simulink model "Vehicle_Model_999_Modular_roll_gradient"  (R2025b)
settings: Solver=ode23tb  StartTime=0.0  StopTime=30  MaxStep=0.001  RelTol=1e-3
values from neighbouring files (symbols this model uses):
  init_r = 0    [Run_this_first.m]
  init_vx = 0    [Run_this_first.m]
  init_vy = 0    [Run_this_first.m]
  Ki_array = zeros(size(Vx_array))    [Torque_vectoring_lookup_table_v3.m]    (also in Torque_vectoring_workspace_lookuptable_v2.m)
  Kp_array = zeros(size(Vx_array))    [Torque_vectoring_workspace_lookuptable_v2.m]
  ku = (lr*m/(cf*(lf+lr))) - (lf*m/(cr*(lf+lr)))    (= -0.000176093739153)    [Torque_vectoring_lookup_table_v3.m]    (also in Torque_vectoring_workspace_lookuptable_v2.m)
  m = Par.m    [LapSim_Endurance_final_ts_v2.m]    (also in Lap_Sim_Final_inverse.m = Par.Mass; Lapsim_Endurance_final_ts.m; New_LapSim_final_ts_v1.m = Par.Mass; Torque_vectoring_lookup_table_v3.m = 270)
  Par = struct()    [Load_vehicle_parameters.m]
  path_Theta = unwrap(atan2(dY, dX))    [New_LapSim_final_ts_v1.m]
  sus_par = struct()    [Load_sus_parameters.m]
  TireData = []    [Lapsim_final_for_app.m]
  V_ref = 45    [Run_this_first.m]
  Vx_array = 1:2:21    [Torque_vectoring_lookup_table_v3.m]    (also in Torque_vectoring_workspace_lookuptable_v2.m = 1:1:21)
undefined symbols (not defined in the file or in its folder): Battery, Brake_Val, ctrl_Brake, ctrl_s, ctrl_Steer, ctrl_Throttle, ctrl_Velocity, HP, Motor, path_X, path_Y, steer_input, Steer_Val, TC_target_slip, Throttle_Val
libraries: simulink x9, autolibshared x3, simulink_extras x2, BatteryEstimators x1
(part 1 of 4)
settings Model: PauseTimes=2  PacingRate=0.001000  Creator=vishal bhujbal  LastModifiedBy=vishal bhujbal
settings SolverCC: ZeroCrossAlgorithm=Adaptive
settings DebuggingCC: AlgebraicLoopMsg=none  IgnoredZcDiagnostic=none

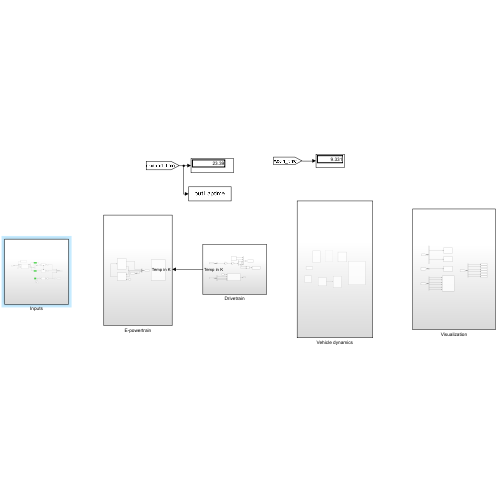
[thumbnail: Simulink's stored preview of the top-level diagram]
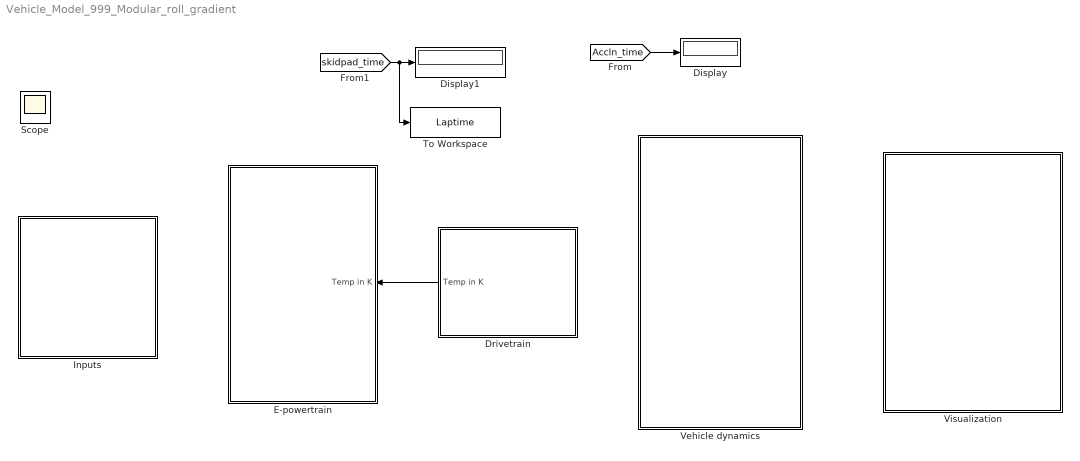
== system Vehicle_Model_999_Modular_roll_gradient ==
  Display : Display
  Display1 : Display
  Drivetrain : Subsystem
      settings: PortSchema="{\"entries\":[{\"content\":{\"sides\":[{\"content\":{\"connectorIds\":[\"Out1\"]},\"type\":\"ConnectorPlacement.EquallySpacedRectSide\",\"uuid\":\"f91cf200-6219-4a1f-80fc-b884c938b97c\"},{\"content\":{\"side\":\"RIGHT\"},\"type\":\"ConnectorPlacement.EquallySpacedRectSide\",\"uuid\":\"1ef2f2a3-0f7e-4e07-a3c9-4fbc06387d99\"},{\"content\":{\"side\":\"TOP\"},\"type\":\"ConnectorPlacement.EquallySpacedRectSide\",\"uuid\":\"4c772986-3ff5-4393-833e-99a2f9c9a16c\"}]},\"type\":\"ConnectorPlacement.EquallySpacedConnector\",\"uuid\":\"ee383106-a54d-4e3a-9b59-9d3772818309\"}],\"packageUris\":[\"http://schema.mathworks.com/mf0/Connector/R2020b\"],\"version\":\"1.0\"}"
  E-powertrain : Subsystem
      settings: PortSchema="{\"entries\":[{\"content\":{\"sides\":[{\"content\":{},\"type\":\"ConnectorPlacement.EquallySpacedRectSide\",\"uuid\":\"2fbe1a29-d7e0-46b2-8acf-c3c60596dfc1\"},{\"content\":{\"connectorIds\":[\"In1\"],\"side\":\"RIGHT\"},\"type\":\"ConnectorPlacement.EquallySpacedRectSide\",\"uuid\":\"5e79f07f-e655-4956-8ef7-fa1f6819f89c\"},{\"content\":{\"side\":\"TOP\"},\"type\":\"ConnectorPlacement.EquallySpacedRectSide\",\"uuid\":\"1ad69596-8b46-43d7-b59f-7fdc3ee385c3\"}]},\"type\":\"ConnectorPlacement.EquallySpacedConnector\",\"uuid\":\"13a1ddb3-f917-41b3-84b0-bd7fb91c78c5\"}],\"packageUris\":[\"http://schema.mathworks.com/mf0/Connector/R2020b\"],\"version\":\"1.0\"}"
  Inputs : Subsystem
  To Workspace : ToWorkspace  VariableName=Laptime  SaveFormat=Timeseries  SampleTime=-1
  Vehicle dynamics : Subsystem
  Visualization : Subsystem
  Scope : Scope
      settings: ActiveDisplayYMinimum=-5.6819269348628578E-5  ActiveDisplayYMaximum=6.3132521498476184E-6  DataLoggingVariableName=ScopeData7
  wires:
  Drivetrain/1(Temp in K) -> E-powertrain/1(Temp in K)
  [Accln_time] -> Display/1
  [skidpad_time] -> To Workspace/1, Display1/1

== system Vehicle_Model_999_Modular_roll_gradient/Drivetrain ==
  Add : Sum
  Bus Selector : BusSelector  OutputSignals=SoC,Omega,I_dc
  Bus Selector1 : BusSelector  OutputSignals=Motor_torque
  Constant : Constant  Value=298
  Demux : Demux  Outputs=2
  Gear Ratio : Gain  Gain=Motor.gear_ratio
  MATLAB Function : MATLAB Function  TreatAsAtomicUnit=on
  Mux : Mux
  Overall Powertrain Efficiency : Gain  Gain=Motor.overall_efficiency
  Thermal : Subsystem
  To Workspace : ToWorkspace  VariableName=Total_wheel_torque  SaveFormat=Timeseries  SampleTime=-1
  Temp in K : Outport
  tag scope: Wheel_torques=global
  wires:
  Bus Selector1/1 -> Gear Ratio/1  "<Motor_torque>"
  Gear Ratio/1 -> Overall Powertrain Efficiency/1
  MATLAB Function/1(T_fl) -> Mux/1
  MATLAB Function/2(T_fr) -> Mux/2
  Demux/1 -> Add/1, Mux/3
  Demux/2 -> Add/2, Mux/4
  Mux/1 -> [Wheel_torques]
  Overall Powertrain Efficiency/1 -> Demux/1
  Thermal/1(Temp in K) -> Temp in K/1
  [Motor_bus] -> Bus Selector/1
  Bus Selector/1 -> Thermal/2(SoC)  "<SoC>"
  Bus Selector/2 -> Thermal/3(Motor speed)  "<Omega>"
  Bus Selector/3 -> Thermal/4(I_dc)  "<I_dc>"
  Constant/1 -> Thermal/1(Ambient Temp)
  [Motor_bus] -> Bus Selector1/1
  Add/1 -> To Workspace/1

== system Vehicle_Model_999_Modular_roll_gradient/E-powertrain ==
  Temp in K : Inport
  Battery Pack : Subsystem
      settings: PortSchema="{\"entries\":[{\"content\":{\"sides\":[{\"content\":{\"connectorIds\":[\"In1\",\"Out2\",\"In2\"]},\"type\":\"ConnectorPlacement.EquallySpacedRectSide\",\"uuid\":\"a12b09be-87e3-41a8-9cce-cb6644b5ba86\"},{\"content\":{\"connectorIds\":[\"Out1\"],\"side\":\"RIGHT\"},\"type\":\"ConnectorPlacement.EquallySpacedRectSide\",\"uuid\":\"19bc61ba-c6fa-40ce-bed9-9c9078ba9fa2\"},{\"content\":{\"side\":\"TOP\"},\"type\":\"ConnectorPlacement.EquallySpacedRectSide\",\"uuid\":\"764d1c28-9cba-450b-a0fd-2f7d4cb2b59a\"}]},\"type\":\"ConnectorPlacement.EquallySpacedConnector\",\"uuid\":\"5b2b37a7-d27f-4738-b8eb-71ceac25d5fc\"}],\"packageUris\":[\"http://schema.mathworks.com/mf0/Connector/R2020b\"],\"version\":\"1.0\"}"
  Bus Creator : BusCreator  Inputs=4
  Bus Selector4 : BusSelector  OutputSignals=Omega
  Motor : Subsystem
  Torque Distribution : Subsystem
  tag scope: Motor_bus=global
  wires:
  Battery Pack/1(V_dc) -> Motor/1(v_dc)
  Motor/1(Motor Torque) -> Bus Creator/1  "Motor_torque"
  Motor/2(I_dc) -> Bus Creator/2, Battery Pack/1(I_dc)  "I_dc"
  Temp in K/1 -> Battery Pack/2(Temp in K)
  Battery Pack/2(SoC) -> Bus Creator/3  "SoC"
  Bus Creator/1 -> [Motor_bus]
  [Wheel_bus] -> Bus Selector4/1
  Bus Selector4/1 -> Bus Creator/4  "<Omega>"

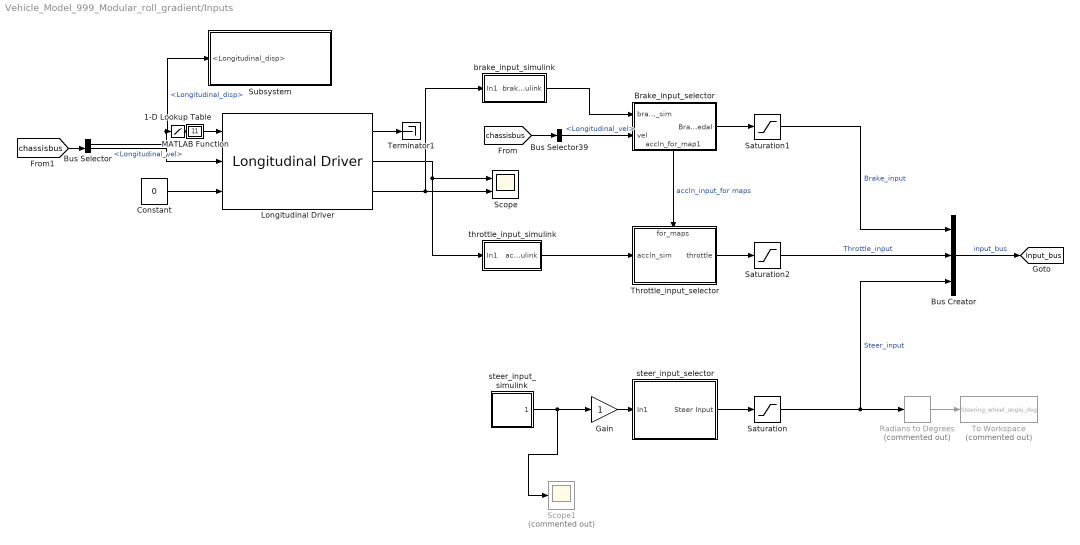
== system Vehicle_Model_999_Modular_roll_gradient/Inputs ==
  1-D Lookup Table : Lookup_n-D  NumberOfTableDimensions=1  BreakpointsForDimension1=ctrl_s  Table=ctrl_Velocity  InternalRulePriority=Speed  RndMeth=Simplest
  Brake_input_selector : Subsystem
      settings: PortSchema="{\"entries\":[{\"content\":{\"sides\":[{\"content\":{\"connectorIds\":[\"In1\",\"In2\"]},\"type\":\"ConnectorPlacement.EquallySpacedRectSide\",\"uuid\":\"eae5282b-8d4e-4a76-acd5-b309529286e8\"},{\"content\":{\"connectorIds\":[\"Out1\"],\"side\":\"RIGHT\"},\"type\":\"ConnectorPlacement.EquallySpacedRectSide\",\"uuid\":\"e88b1ae5-ebac-4dec-84e3-4990dfef2a20\"},{\"content\":{\"side\":\"TOP\"},\"type\":\"ConnectorPlacement.EquallySpacedRectSide\",\"uuid\":\"953e68b4-cb24-4ebf-9e87-e8908532a5e9\"},{\"content\":{\"connectorIds\":[\"Out2\"],\"side\":\"BOTTOM\"},\"type\":\"ConnectorPlacement.EquallySpacedRectSide\",\"uuid\":\"cb4e4aaa-ddd9-4948-8132-cd5bc6a16c6f\"}]},\"type\":\"ConnectorPlacement.EquallySpacedConnector\",\"uuid\":\"c57fd576-21a2-411a-8f11-bf01f4b27bc3\"}],\"packageUris\":[\"http://schema.mathworks.com/mf0/Connector/R2020b\"],\"version\":\"1.0\"}"
  Bus Creator : BusCreator  Inputs=3
  Bus Selector : BusSelector  OutputSignals=Longitudinal_disp,Longitudinal_vel
  Bus Selector39 : BusSelector  OutputSignals=Longitudinal_vel
  Constant : Constant  Value=0
  Gain : Gain
  Longitudinal Driver : autolibshared/Longitudinal Driver  extAccelOvr=off  extDecelOvr=off  extAccelHld=off  extDecelHld=off  extAccelZero=off  extDecelZero=off  cntrlType=PI  shftType=None  velUnits=m/s  gearOut=off  Kp=13.2353  Ki=5.00045  Kff=0.15  Kg=0  VehVelVec=[0 100]  KffVec=[.1 .1]  KpVec=[10 10]  KiVec=[5 5]  KgVec=[0 0]  m=1500  Kpt=3000  tau=.1  L=2  aR=200  bR=2.5  cR=.5  g=9.81  vnom=5  Kaw=1  tauerr=.01  tauPt=2  GearInit=0  tShift=.1  pdlVec=[0.1 0.4 0.5 0.9]  upShftTbl=[-1 12.9375 26.4375 39.9375 51.18749999999999 62.4375 72.84375 83.25;-1 16.3125 29.8125 43.3125 54.5624 65.8125 76.78125 87.75;-1 19.6875 33.1875 46.68749999999999 57.9375 69.1875 80.71875 92.25;-1 33 52.5 77.25 100.5 138.75 161.875 185]  dwnShftTbl=[1 9.5625 23.0625 36.5625 47.8125 59.0625 68.90625 78.75;1 12.9375 26.4375 39.9375 51.18749999999999 62.4375 72.84375 83.25;1 16.3125 29.8125 43.3125 54.562499 65.8125 76.78125 87.75;1 19.6875 33.1875 46.68749999999999 57.9375 69.1875 80.71875 92.25]  tClutch=.5  tRev=.5  tPark=120  aMode=2  UpGearVec="[0  1  2  3  4  5  6  7]"  DownGearVec="[1  2  3  4  5  6  7  8]"
      settings: LibrarySourceBlock=vehdynlibdriver/Longitudinal Driver
  MATLAB Function : MATLAB Function  TreatAsAtomicUnit=on
  Radians to Degrees : simulink_extras/Transformations/Radians to Degrees  Commented=on
  Saturation : Saturate  UpperLimit=pi/6  LowerLimit=-pi/6
  Saturation1 : Saturate  UpperLimit=1  LowerLimit=0
  Saturation2 : Saturate  UpperLimit=1  LowerLimit=0
  Scope : Scope  NumInputPorts=2
      settings: ActiveDisplayYMinimum=-0.12499999999999997  ActiveDisplayYMaximum=1.125  DataLoggingVariableName=ScopeData9
  Scope1 : Scope  Commented=on
      settings: ActiveDisplayYMinimum=-0.21672639126737681  ActiveDisplayYMaximum=0.21672588045733382  DataLoggingVariableName=ScopeData14
  Subsystem : Subsystem
  Terminator1 : Terminator
  Throttle_input_selector : Subsystem
      settings: PortSchema="{\"entries\":[{\"content\":{\"sides\":[{\"content\":{\"connectorIds\":[\"In1\"]},\"type\":\"ConnectorPlacement.EquallySpacedRectSide\",\"uuid\":\"91e59d49-26fd-4266-b297-7cd1b1ce02c9\"},{\"content\":{\"connectorIds\":[\"Out1\"],\"side\":\"RIGHT\"},\"type\":\"ConnectorPlacement.EquallySpacedRectSide\",\"uuid\":\"6279f554-8ceb-423b-aff4-2d71feb4a43a\"},{\"content\":{\"connectorIds\":[\"In2\"],\"side\":\"TOP\"},\"type\":\"ConnectorPlacement.EquallySpacedRectSide\",\"uuid\":\"41f52c32-a07b-4398-ae75-202afa1bbaca\"}]},\"type\":\"ConnectorPlacement.EquallySpacedConnector\",\"uuid\":\"9d03091e-cc24-4a85-a828-51493ad70cf1\"}],\"packageUris\":[\"http://schema.mathworks.com/mf0/Connector/R2020b\"],\"version\":\"1.0\"}"
  To Workspace : ToWorkspace  Commented=on  VariableName=Steering_wheel_angle_deg  SaveFormat=Timeseries  SampleTime=-1
  brake_input_simulink : Subsystem
  steer_input_selector : Subsystem
  steer_input_simulink : Subsystem
  throttle_input_simulink : Subsystem
  tag scope: Input_bus=global
  wires:
  Throttle_input_selector/1(throttle) -> Saturation2/1
  throttle_input_simulink/1(accln_simulink) -> Throttle_input_selector/1(accln_sim)
  Brake_input_selector/2(accln_for_map1) -> Throttle_input_selector/2(for_maps)  "accln_input_for maps"
  Bus Selector39/1 -> Brake_input_selector/2(vel)  "<Longitudinal_vel>"
  Brake_input_selector/1(Brake pedal) -> Saturation1/1
  brake_input_simulink/1(brake_simulink) -> Brake_input_selector/1(brake_sim)
  steer_input_simulink/1(cmd_str) -> Scope1/1, Gain/1
  steer_input_selector/1(Steer Input) -> Saturation/1
  Bus Creator/1 -> [Input_bus]  "input_bus"
  Saturation/1 -> Radians to Degrees/1, Bus Creator/3  "Steer_input"
  Saturation1/1 -> Bus Creator/1  "Brake_input"
  Saturation2/1 -> Bus Creator/2  "Throttle_input"
  [chassisbus] -> Bus Selector39/1
  Radians to Degrees/1 -> To Workspace/1
  [chassisbus] -> Bus Selector/1
  Bus Selector/2 -> Longitudinal Driver/2  "<Longitudinal_vel>"
  Constant/1 -> Longitudinal Driver/3
  Bus Selector/1 -> Subsystem/1(<Longitudinal_disp>), 1-D Lookup Table/1  "<Longitudinal_disp>"
  Longitudinal Driver/2 -> throttle_input_simulink/1(In1), Scope/1
  Longitudinal Driver/1 -> Terminator1/1
  MATLAB Function/1(y) -> Longitudinal Driver/1
  Longitudinal Driver/3 -> brake_input_simulink/1(In1), Scope/2
  Gain/1 -> steer_input_selector/1(In1)
  1-D Lookup Table/1 -> MATLAB Function/1(ideal_ref_vel)

== system Vehicle_Model_999_Modular_roll_gradient/Vehicle dynamics ==
  Brakes : Subsystem
  Force and Torque Equilibrium : Subsystem
  "Fx, Fy calculations" : Subsystem  Commented=on
  "Fx, Fy calculations with grip limit" : Subsystem
  Rolling and Drag forces : Subsystem
  Steering : Subsystem
  Suspension : Subsystem
  Wheel_dynamics : Subsystem
  wires:
  Wheel_dynamics/1(Omega1) -> Suspension/1(Omega)

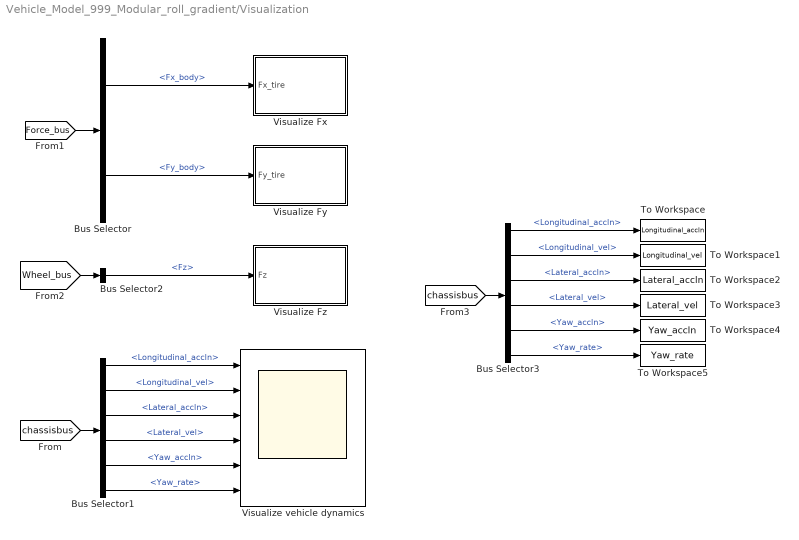
== system Vehicle_Model_999_Modular_roll_gradient/Visualization ==
  Bus Selector : BusSelector  OutputSignals=Fx_body,Fy_body
  Bus Selector1 : BusSelector  OutputSignals=Longitudinal_accln,Longitudinal_vel,Lateral_accln,Lateral_vel,Yaw_accln,Yaw_rate
  Bus Selector2 : BusSelector  OutputSignals=Fz
  Bus Selector3 : BusSelector  OutputSignals=Longitudinal_accln,Longitudinal_vel,Lateral_accln,Lateral_vel,Yaw_accln,Yaw_rate
  To Workspace : ToWorkspace  VariableName=Longitudinal_accln  SaveFormat=Timeseries  SampleTime=-1
  To Workspace1 : ToWorkspace  VariableName=Longitudinal_vel  SaveFormat=Timeseries  SampleTime=-1
  To Workspace2 : ToWorkspace  VariableName=Lateral_accln  SaveFormat=Timeseries  SampleTime=-1
  To Workspace3 : ToWorkspace  VariableName=Lateral_vel  SaveFormat=Timeseries  SampleTime=-1
  To Workspace4 : ToWorkspace  VariableName=Yaw_accln  SaveFormat=Timeseries  SampleTime=-1
  To Workspace5 : ToWorkspace  VariableName=Yaw_rate  SaveFormat=Timeseries  SampleTime=-1
  Visualize Fx : Subsystem
  Visualize Fy : Subsystem
  Visualize Fz : Subsystem
  Visualize vehicle dynamics : Scope  NumInputPorts=6
      settings: ActiveDisplayYMinimum=-11.262828862578662  ActiveDisplayYMaximum=8.2206676714982336
  wires:
  [Force_bus] -> Bus Selector/1
  [chassisbus] -> Bus Selector1/1
  Bus Selector1/1 -> Visualize vehicle dynamics/1  "<Longitudinal_accln>"
  Bus Selector1/2 -> Visualize vehicle dynamics/2  "<Longitudinal_vel>"
  Bus Selector1/3 -> Visualize vehicle dynamics/3  "<Lateral_accln>"
  Bus Selector1/4 -> Visualize vehicle dynamics/4  "<Lateral_vel>"
  Bus Selector1/5 -> Visualize vehicle dynamics/5  "<Yaw_accln>"
  Bus Selector/1 -> Visualize Fx/1(Fx_tire)  "<Fx_body>"
  [Wheel_bus] -> Bus Selector2/1
  Bus Selector2/1 -> Visualize Fz/1(Fz)  "<Fz>"
  Bus Selector3/5 -> To Workspace4/1  "<Yaw_accln>"
  Bus Selector3/4 -> To Workspace3/1  "<Lateral_vel>"
  Bus Selector3/3 -> To Workspace2/1  "<Lateral_accln>"
  Bus Selector3/2 -> To Workspace1/1  "<Longitudinal_vel>"
  Bus Selector3/1 -> To Workspace/1  "<Longitudinal_accln>"
  [chassisbus] -> Bus Selector3/1
  Bus Selector/2 -> Visualize Fy/1(Fy_tire)  "<Fy_body>"
  Bus Selector3/6 -> To Workspace5/1  "<Yaw_rate>"
  Bus Selector1/6 -> Visualize vehicle dynamics/6  "<Yaw_rate>"

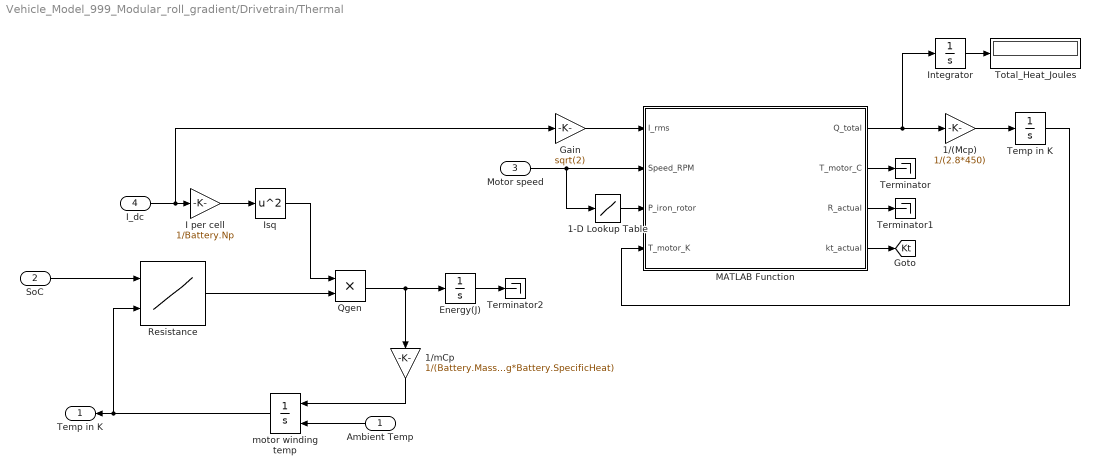
== system Vehicle_Model_999_Modular_roll_gradient/Drivetrain/Thermal ==
  Ambient Temp : Inport
  SoC : Inport  Port=2
  Motor speed : Inport  Port=3
  I_dc : Inport  Port=4
  1-D Lookup Table : Lookup_n-D  NumberOfTableDimensions=1  BreakpointsForDimension1=[0 5000 10000 12500 15000 20000]  Table=[0 105 230 300 310 315]  InternalRulePriority=Speed  RndMeth=Simplest
  1/(Mcp) : Gain  Gain=1/(2.8*450)
  1/mCp : Gain  Gain=1/(Battery.Mass_kg*Battery.SpecificHeat)
  Energy(J) : Integrator
  Gain : Gain  Gain=sqrt(2)
  I per cell : Gain  Gain=1/Battery.Np
  Integrator : Integrator
  Isq : Math  Operator=square
  MATLAB Function : MATLAB Function  TreatAsAtomicUnit=on
  Qgen : Product
  Resistance : Lookup_n-D  BreakpointsForDimension1=Battery.SoC_vec  BreakpointsForDimension2=Battery.T_vec  Table=Battery.R0_map+Battery.R1_map  InternalRulePriority=Speed  RndMeth=Simplest
      settings: InputPortMap=u0,u1
  "Temp in K " : Integrator  InitialCondition=293.15  LimitOutput=on  UpperSaturationLimit=423.15  LowerSaturationLimit=293.15
  Terminator : Terminator
  Terminator1 : Terminator
  Terminator2 : Terminator
  Total_Heat_Joules : Display
  motor winding temp : Integrator  InitialConditionSource=external  InitialCondition=298.15
  Temp in K : Outport
  tag scope: Kt=global
  wires:
  Qgen/1 -> Energy(J)/1, 1/mCp/1
  Resistance/1 -> Qgen/2
  motor winding temp/1 -> Temp in K/1, Resistance/2
  I per cell/1 -> Isq/1
  1/mCp/1 -> motor winding temp/1
  Isq/1 -> Qgen/1
  SoC/1 -> Resistance/1
  Ambient Temp/1 -> motor winding temp/2
  1/(Mcp)/1 -> "Temp in K "/1
  Motor speed/1 -> MATLAB Function/2(Speed_RPM), 1-D Lookup Table/1
  I_dc/1 -> Gain/1, I per cell/1
  1-D Lookup Table/1 -> MATLAB Function/3(P_iron_rotor)
  MATLAB Function/4(kt_actual) -> [Kt]
  Integrator/1 -> Total_Heat_Joules/1
  MATLAB Function/1(Q_total) -> Integrator/1, 1/(Mcp)/1
  Gain/1 -> MATLAB Function/1(I_rms)
  "Temp in K "/1 -> MATLAB Function/4(T_motor_K)
  MATLAB Function/2(T_motor_C) -> Terminator/1
  MATLAB Function/3(R_actual) -> Terminator1/1
  Energy(J)/1 -> Terminator2/1

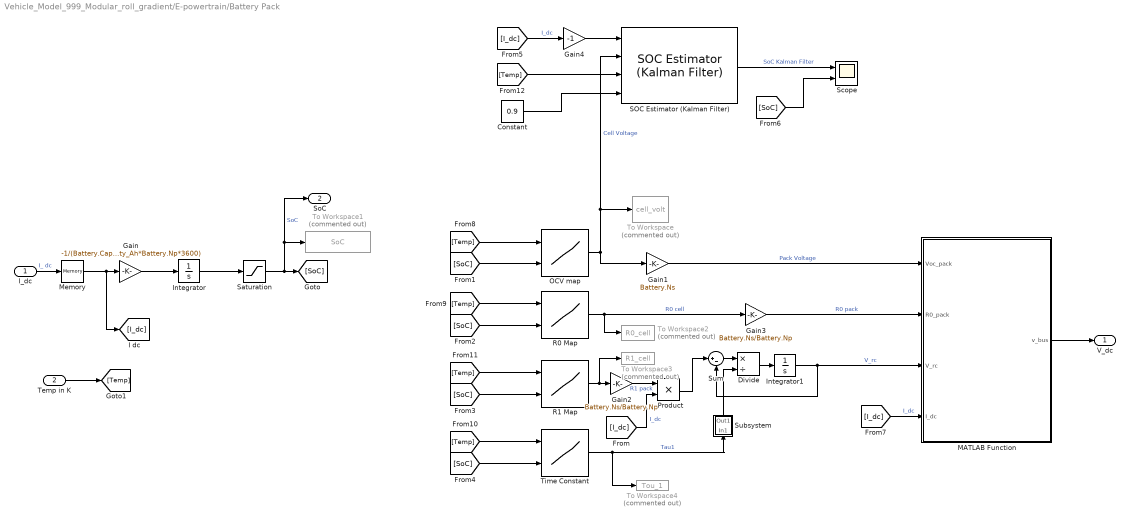
== system Vehicle_Model_999_Modular_roll_gradient/E-powertrain/Battery Pack ==
  I_dc : Inport
  Temp in K : Inport  Port=2
  Constant : Constant  Value=0.9
  Divide : Product  Inputs=*/
  Gain : Gain  Gain=-1/(Battery.Capacity_Ah*Battery.Np*3600)
  Gain1 : Gain  Gain=Battery.Ns
  Gain2 : Gain  Gain=Battery.Ns/Battery.Np
  Gain3 : Gain  Gain=Battery.Ns/Battery.Np
  Gain4 : Gain  Gain=-1
  Integrator : Integrator  InitialCondition=1
  Integrator1 : Integrator
  MATLAB Function : MATLAB Function  TreatAsAtomicUnit=on
  Memory : Memory
  OCV map : Lookup_n-D  BreakpointsForDimension1=Battery.T_vec  BreakpointsForDimension2=Battery.SoC_vec  Table=Battery.OCV_map'  InternalRulePriority=Speed  RndMeth=Simplest
      settings: InputPortMap=u0,u1
  Product : Product
  R0 Map : Lookup_n-D  BreakpointsForDimension1=Battery.T_vec  BreakpointsForDimension2=Battery.SoC_vec  Table=Battery.R0_map'  InternalRulePriority=Speed  RndMeth=Simplest
      settings: InputPortMap=u0,u1
  R1 Map : Lookup_n-D  BreakpointsForDimension1=Battery.T_vec  BreakpointsForDimension2=Battery.SoC_vec  Table=Battery.R1_map'  InternalRulePriority=Speed  RndMeth=Simplest
      settings: InputPortMap=u0,u1
  SOC Estimator (Kalman Filter) : BatteryEstimators/SOC Estimator (Kalman Filter)  CurrentInputPartition=off  filterType=Extended Kalman filter  alpha=1  beta=2  kappa=0  Q=|  Q_2RC=|  R=0.1  P0=[1e-5 0; 0 1]  P0_2RC=[1e-5 0 0; 0 1 0;0 0 1]  Ts=1  chargeDynamics=One time-constant dynamics  SOC_vec=[0 0.1 0.25 0.5 0.75 0.9 1]  T_vec=[278 293 313]  R0_mat=[0.0117 0.0085 0.009;0.011 0.0085 0.009;0.0114 0.0087 0.0092;0.0107 0.0082 0.0088;0.0107 0.0083 0.0091;0.0113 0.0085 0.0089;0.0116 0.0085 0.0089]  R1_mat=[0.0109 0.0029 0.0013;0.0069 0.0024 0.0012;0.0047 0.0026 0.0013;0.0034 0.0016 0.001;0.0033 0.0023 0.0014;0.0033 0.0018 0.0011;0.0028 0.0017 0.0011]  tau1_mat=[20 36 39;31 45 39;109 105 61;36 29 26;59 77 67;40 33 29;25 39 33]  R2_mat=[.0109, .0029, .0013; .0069, .0024, .0012; .0047, .0026, .0013; .0034, .0016, .001; .0033, .0023, .0014; .0033, .0018, .0011; .0028, .0017, .0011]  tau2_mat=[20, 36, 39; 31, 45, 39; 109, 105, 61; 36, 29, 26; 59, 77, 67; 40, 33, 29; 25, 39, 33]  V0_mat=[3.49 3.5 3.51;3.55 3.57 3.56;3.62 3.63 3.64;3.71 3.71 3.72;3.91 3.93 3.94;4.07 4.08 4.08;4.19 4.19 4.19]  AH=4.493  DataType=Inherit: auto
      Q=|
      | [1e-6 0;
      | 0 1e-6]
      Q_2RC=|
      | [1e-6 0 0;
      | 0 1e-6 0; 0 0 1e-6]
  Saturation : Saturate  UpperLimit=1  LowerLimit=0
  Scope : Scope  NumInputPorts=2
      settings: ActiveDisplayYMinimum=0.87799639857607525  ActiveDisplayYMaximum=0.90245265023893717  DataLoggingVariableName=ScopeData8
  Subsystem : Subsystem
  Sum : Sum  Inputs=|+-
  Time Constant : Lookup_n-D  BreakpointsForDimension1=Battery.T_vec  BreakpointsForDimension2=Battery.SoC_vec  Table=Battery.Tau_map'  InternalRulePriority=Speed  RndMeth=Simplest
      settings: InputPortMap=u0,u1
  To Workspace : ToWorkspace  Commented=on  VariableName=cell_volt  SaveFormat=Timeseries  SampleTime=-1
  To Workspace1 : ToWorkspace  Commented=on  VariableName=SoC  SaveFormat=Timeseries  SampleTime=-1
  To Workspace2 : ToWorkspace  Commented=on  VariableName=R0_cell  SaveFormat=Timeseries  SampleTime=-1
  To Workspace3 : ToWorkspace  Commented=on  VariableName=R1_cell  SaveFormat=Timeseries  SampleTime=-1
  To Workspace4 : ToWorkspace  Commented=on  VariableName=Tou_1  SaveFormat=Timeseries  SampleTime=-1
  V_dc : Outport
  SoC : Outport  Port=2
  wires:
  Gain4/1 -> SOC Estimator (Kalman Filter)/1
  Memory/1 -> Gain/1, [I_dc]
  [Temp] -> SOC Estimator (Kalman Filter)/3
  [Temp] -> Time Constant/1
  [Temp] -> R1 Map/1
  [Temp] -> R0 Map/1
  [Temp] -> OCV map/1
  Temp in K/1 -> [Temp]
  [I_dc] -> MATLAB Function/4(I_dc)  "I_dc"
  [SoC] -> Scope/2
  [I_dc] -> Gain4/1  "I_dc"
  [SoC] -> OCV map/2
  [SoC] -> R0 Map/2
  [SoC] -> R1 Map/2
  [SoC] -> Time Constant/2
  Saturation/1 -> [SoC], SoC/1, To Workspace1/1  "SoC"
  [I_dc] -> Product/2  "I_dc"
  MATLAB Function/1(v_bus) -> V_dc/1
  SOC Estimator (Kalman Filter)/1 -> Scope/1  "SoC Kalman Filter"
  Constant/1 -> SOC Estimator (Kalman Filter)/4
  Divide/1 -> Integrator1/1
  Time Constant/1 -> Subsystem/1(In1), To Workspace4/1  "Tau1"
  Sum/1 -> Divide/1
  Integrator1/1 -> Sum/2, MATLAB Function/3(V_rc)  "V_rc"
  Product/1 -> Sum/1
  Gain2/1 -> Product/1  "R1 pack"
  Gain3/1 -> MATLAB Function/2(R0_pack)  "R0 pack"
  R0 Map/1 -> Gain3/1, To Workspace2/1  "R0 cell"
  R1 Map/1 -> Gain2/1, To Workspace3/1
  Gain1/1 -> MATLAB Function/1(Voc_pack)  "Pack Voltage"
  OCV map/1 -> Gain1/1, To Workspace/1, SOC Estimator (Kalman Filter)/2  "Cell Voltage"
  Integrator/1 -> Saturation/1
  Gain/1 -> Integrator/1
  I_dc/1 -> Memory/1  "I_ dc"
  Subsystem/1(Out1) -> Divide/2

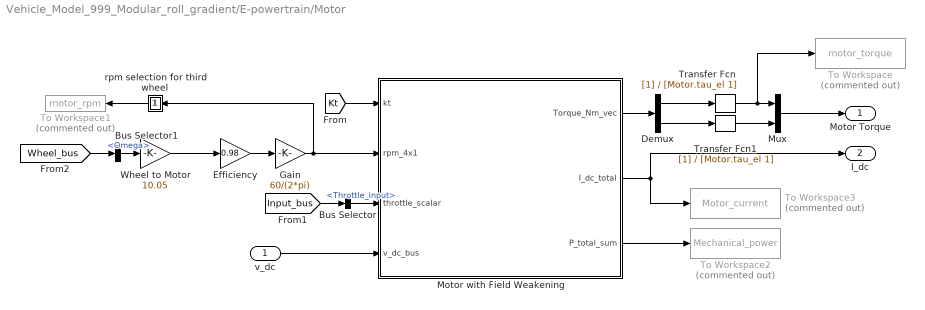
== system Vehicle_Model_999_Modular_roll_gradient/E-powertrain/Motor ==
  v_dc : Inport
  Bus Selector : BusSelector  OutputSignals=Throttle_input
  Bus Selector1 : BusSelector  OutputSignals=Omega
  Demux : Demux  Outputs=2
  Efficiency : Gain  Gain=0.98
  Gain : Gain  Gain=60/(2*pi)
  Motor with Field Weakening : MATLAB Function  TreatAsAtomicUnit=on
  Mux : Mux  Inputs=2
  To Workspace : ToWorkspace  Commented=on  VariableName=motor_torque  SaveFormat=Timeseries  SampleTime=-1
  To Workspace1 : ToWorkspace  Commented=on  VariableName=motor_rpm  SaveFormat=Timeseries  SampleTime=-1
  To Workspace2 : ToWorkspace  Commented=on  VariableName=Mechanical_power  SaveFormat=Timeseries  SampleTime=-1
  To Workspace3 : ToWorkspace  Commented=on  VariableName=Motor_current  SaveFormat=Timeseries  SampleTime=-1
  Transfer Fcn : TransferFcn  Denominator=[Motor.tau_el 1]
  Transfer Fcn1 : TransferFcn  Denominator=[Motor.tau_el 1]
  Wheel to Motor : Gain  Gain=10.05
  rpm selection for third wheel : MATLAB Function  TreatAsAtomicUnit=on
  Motor Torque : Outport
  I_dc : Outport  Port=2
  wires:
  rpm selection for third wheel/1(y) -> To Workspace1/1
  Motor with Field Weakening/3(P_total_sum) -> To Workspace2/1
  Mux/1 -> Motor Torque/1
  Transfer Fcn/1 -> Mux/1, To Workspace/1
  Demux/2 -> Transfer Fcn1/1
  Transfer Fcn1/1 -> Mux/2
  Demux/1 -> Transfer Fcn/1
  Motor with Field Weakening/1(Torque_Nm_vec) -> Demux/1
  Motor with Field Weakening/2(I_dc_total) -> To Workspace3/1, I_dc/1
  Efficiency/1 -> Gain/1
  Wheel to Motor/1 -> Efficiency/1
  v_dc/1 -> Motor with Field Weakening/4(v_dc_bus)
  [Kt] -> Motor with Field Weakening/1(kt)
  [Input_bus] -> Bus Selector/1
  Bus Selector/1 -> Motor with Field Weakening/3(throttle_scalar)  "<Throttle_input>"
  [Wheel_bus] -> Bus Selector1/1
  Bus Selector1/1 -> Wheel to Motor/1  "<Omega>"
  Gain/1 -> rpm selection for third wheel/1(u), Motor with Field Weakening/2(rpm_4x1)

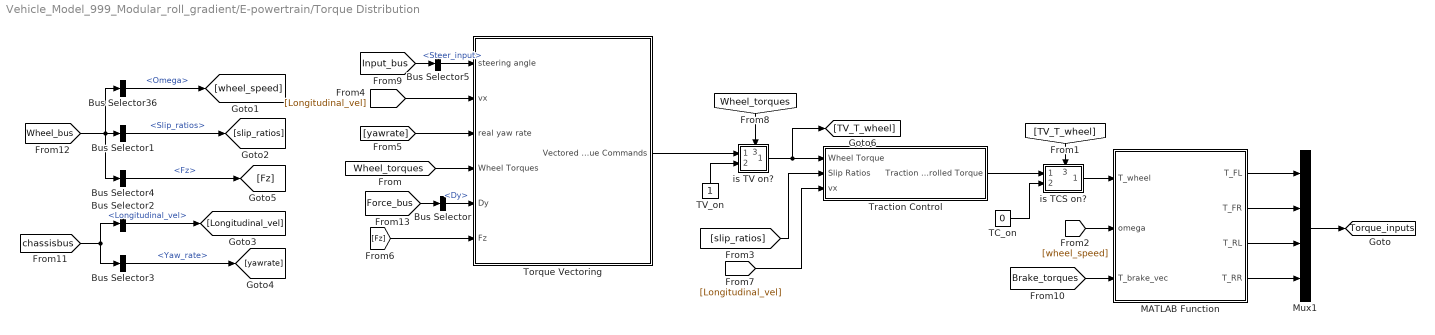
== system Vehicle_Model_999_Modular_roll_gradient/E-powertrain/Torque Distribution ==
  Bus Selector : BusSelector  OutputSignals=Dy
  Bus Selector1 : BusSelector  OutputSignals=Slip_ratios
  Bus Selector2 : BusSelector  OutputSignals=Longitudinal_vel
  Bus Selector3 : BusSelector  OutputSignals=Yaw_rate
  Bus Selector36 : BusSelector  OutputSignals=Omega
  Bus Selector4 : BusSelector  OutputSignals=Fz
  Bus Selector5 : BusSelector  OutputSignals=Steer_input
  MATLAB Function : MATLAB Function  TreatAsAtomicUnit=on
  Mux1 : Mux
  TC_on : Constant  Value=0
  TV_on : Constant
  Torque Vectoring : Subsystem
  Traction Control : Subsystem
  is TCS on? : Subsystem
      settings: PortSchema="{\"entries\":[{\"content\":{\"sides\":[{\"content\":{\"connectorIds\":[\"In1\",\"In2\"]},\"type\":\"ConnectorPlacement.EquallySpacedRectSide\",\"uuid\":\"dc8df3c8-a53f-4de0-9df1-c7ce6985ad6f\"},{\"content\":{\"connectorIds\":[\"Out1\"],\"side\":\"RIGHT\"},\"type\":\"ConnectorPlacement.EquallySpacedRectSide\",\"uuid\":\"042501be-c855-4a6a-885a-a96d559db999\"},{\"content\":{\"connectorIds\":[\"In3\"],\"side\":\"TOP\"},\"type\":\"ConnectorPlacement.EquallySpacedRectSide\",\"uuid\":\"e6b24d4f-1e31-4513-950e-4f31e3010837\"}]},\"type\":\"ConnectorPlacement.EquallySpacedConnector\",\"uuid\":\"efc7ad52-73a3-41d4-9bb0-a43132bb4628\"}],\"packageUris\":[\"http://schema.mathworks.com/mf0/Connector/R2020b\"],\"version\":\"1.0\"}"
  is TV on? : Subsystem
      settings: PortSchema="{\"entries\":[{\"content\":{\"sides\":[{\"content\":{\"connectorIds\":[\"In1\",\"In2\"]},\"type\":\"ConnectorPlacement.EquallySpacedRectSide\",\"uuid\":\"dc8df3c8-a53f-4de0-9df1-c7ce6985ad6f\"},{\"content\":{\"connectorIds\":[\"Out1\"],\"side\":\"RIGHT\"},\"type\":\"ConnectorPlacement.EquallySpacedRectSide\",\"uuid\":\"042501be-c855-4a6a-885a-a96d559db999\"},{\"content\":{\"connectorIds\":[\"In3\"],\"side\":\"TOP\"},\"type\":\"ConnectorPlacement.EquallySpacedRectSide\",\"uuid\":\"e6b24d4f-1e31-4513-950e-4f31e3010837\"},{\"content\":{\"side\":\"BOTTOM\"},\"type\":\"ConnectorPlacement.EquallySpacedRectSide\",\"uuid\":\"10630930-7341-43aa-b9d4-dad8f31a30ac\"}]},\"type\":\"ConnectorPlacement.EquallySpacedConnector\",\"uuid\":\"efc7ad52-73a3-41d4-9bb0-a43132bb4628\"}],\"packageUris\":[\"http://schema.mathworks.com/mf0/Connector/R2020b\"],\"version\":\"1.0\"}"
  tag scope: Torque_inputs=global
  wires:
  [Brake_torques] -> MATLAB Function/3(T_brake_vec)
  MATLAB Function/1(T_FL) -> Mux1/1
  MATLAB Function/2(T_FR) -> Mux1/2
  MATLAB Function/3(T_RL) -> Mux1/3
  MATLAB Function/4(T_RR) -> Mux1/4
  Mux1/1 -> [Torque_inputs]
  [Wheel_bus] -> Bus Selector36/1, Bus Selector4/1, Bus Selector1/1
  [chassisbus] -> Bus Selector3/1, Bus Selector2/1
  [Wheel_torques] -> Torque Vectoring/4(Wheel Torques)
  Bus Selector36/1 -> [wheel_speed]  "<Omega>"
  [wheel_speed] -> MATLAB Function/2(omega)
  Bus Selector1/1 -> [slip_ratios]  "<Slip_ratios>"
  [slip_ratios] -> Traction Control/2(Slip Ratios)
  [Longitudinal_vel] -> Torque Vectoring/2(vx)
  Bus Selector2/1 -> [Longitudinal_vel]  "<Longitudinal_vel>"
  Bus Selector3/1 -> [yawrate]  "<Yaw_rate>"
  [yawrate] -> Torque Vectoring/3(real yaw rate)
  is TCS on?/1(torque_output) -> MATLAB Function/1(T_wheel)
  Bus Selector4/1 -> [Fz]  "<Fz>"
  [Fz] -> Torque Vectoring/6(Fz)
  [Longitudinal_vel] -> Traction Control/3(vx)
  Torque Vectoring/1(Vectored Torque Commands) -> is TV on?/1(vectored_torque)
  is TV on?/1(torque_output) -> Traction Control/1(Wheel Torque), [TV_T_wheel]
  [Wheel_torques] -> is TV on?/3(wheel_torque)
  Traction Control/1(Traction Controlled Torque) -> is TCS on?/1(traction_controlled_torque)
  [TV_T_wheel] -> is TCS on?/3(TV_T_wheel)
  TV_on/1 -> is TV on?/2(In1)
  [Input_bus] -> Bus Selector5/1
  Bus Selector5/1 -> Torque Vectoring/1(steering angle)  "<Steer_input>"
  [Force_bus] -> Bus Selector/1
  Bus Selector/1 -> Torque Vectoring/5(Dy)  "<Dy>"
  TC_on/1 -> is TCS on?/2(In1)

== system Vehicle_Model_999_Modular_roll_gradient/Inputs/Brake_input_selector ==
  brake_sim : Inport
  vel : Inport  Port=2
  Brake Variant Subsystem : Subsystem  Variant=on
  Brake pedal : Outport
  accln_for_map1 : Outport  Port=2
  wires:
  Brake Variant Subsystem/1(brake_input) -> Brake pedal/1
  brake_sim/1 -> Brake Variant Subsystem/1(brake_sim)
  vel/1 -> Brake Variant Subsystem/2(vel)
  Brake Variant Subsystem/2(accln) -> accln_for_map1/1

== system Vehicle_Model_999_Modular_roll_gradient/Inputs/Subsystem ==
  <Longitudinal_disp> : Inport
  Clock : Clock
  Compare To Constant : simulink/Logic and Bit Operations/Compare To Constant  relop=>=  const=239  OutDataTypeStr=boolean
  Compare To Constant1 : simulink/Logic and Bit Operations/Compare To Constant  relop=>=  const=10  OutDataTypeStr=boolean
  Compare To Constant2 : simulink/Logic and Bit Operations/Compare To Constant  Commented=on  relop=>=  const=max(ctrl_s)-20.8668-9.8234-7.5  OutDataTypeStr=boolean
  Stop Simulation : Stop
  Subtract : Sum  Inputs=-+
  To Workspace1 : ToWorkspace  VariableName=t2  SaveFormat=Timeseries  SampleTime=-1
  To Workspace2 : ToWorkspace  VariableName=t1  SaveFormat=Timeseries  SampleTime=-1
  Triggered Subsystem : Subsystem  TreatAsAtomicUnit=on
  Triggered Subsystem1 : Subsystem  TreatAsAtomicUnit=on
  Triggered Subsystem2 : Subsystem  TreatAsAtomicUnit=on
  tag scope: skidpad_time=global
  wires:
  Compare To Constant1/1 -> Triggered Subsystem1/Trigger
  Triggered Subsystem/1(Out1) -> Subtract/2, To Workspace1/1  "t2"
  Clock/1 -> Triggered Subsystem1/1(In1), Triggered Subsystem/1(In1)
  <Longitudinal_disp>/1 -> Compare To Constant/1, Compare To Constant1/1
  Triggered Subsystem1/1(Out1) -> Subtract/1, To Workspace2/1  "t1"
  Compare To Constant/1 -> Stop Simulation/1, Triggered Subsystem2/Trigger, Triggered Subsystem/Trigger
  Triggered Subsystem2/1(Out1) -> [skidpad_time]  "t2"
  Subtract/1 -> Triggered Subsystem2/1(In1)

== system Vehicle_Model_999_Modular_roll_gradient/Inputs/Throttle_input_selector ==
  accln_sim : Inport
  for_maps : Inport  Port=2
  Saturation : Saturate  UpperLimit=1  LowerLimit=0
  Throttle Variant Subsystem : Subsystem  Variant=on
  throttle : Outport
  wires:
  Throttle Variant Subsystem/1(throttle) -> Saturation/1
  for_maps/1 -> Throttle Variant Subsystem/2(accln_input_for_map1)
  accln_sim/1 -> Throttle Variant Subsystem/1(accln)
  Saturation/1 -> throttle/1

== system Vehicle_Model_999_Modular_roll_gradient/Inputs/brake_input_simulink ==
  In1 : Inport
  1-D Lookup Table : Lookup_n-D  Commented=on  NumberOfTableDimensions=1  BreakpointsForDimension1=ctrl_s  Table=ctrl_Brake  InternalRulePriority=Speed  RndMeth=Simplest
  Bus Selector : BusSelector  Commented=on  OutputSignals=Longitudinal_disp
  From : From  Commented=on  GotoTag=chassisbus  TagVisibility=global
  brake_simulink : Outport
  wires:
  From/1 -> Bus Selector/1
  Bus Selector/1 -> 1-D Lookup Table/1  "<Longitudinal_disp>"
  In1/1 -> brake_simulink/1

== system Vehicle_Model_999_Modular_roll_gradient/Inputs/steer_input_selector ==
  In1 : Inport
  Steering Variant Subsystem : Subsystem  Variant=on
  Steer Input : Outport
  wires:
  Steering Variant Subsystem/1(Steer Input) -> Steer Input/1
  In1/1 -> Steering Variant Subsystem/1(In1)

== system Vehicle_Model_999_Modular_roll_gradient/Inputs/steer_input_simulink ==
  1-D Lookup Table : Lookup_n-D  NumberOfTableDimensions=1  BreakpointsForDimension1=ctrl_s  Table=ctrl_Steer  InternalRulePriority=Speed  RndMeth=Simplest
  1-D Lookup Table2 : Lookup_n-D  Commented=on  NumberOfTableDimensions=1  BreakpointsForDimension1=ctrl_s  Table=path_Y  InternalRulePriority=Speed  RndMeth=Simplest
  1-D Lookup Table3 : Lookup_n-D  Commented=on  NumberOfTableDimensions=1  BreakpointsForDimension1=ctrl_s  Table=path_X  InternalRulePriority=Speed  RndMeth=Simplest
  1-D Lookup Table4 : Lookup_n-D  Commented=on  NumberOfTableDimensions=1  BreakpointsForDimension1=ctrl_s  Table=path_Theta  InternalRulePriority=Speed  RndMeth=Simplest
  Add : Sum
  Bus Selector : BusSelector  OutputSignals=Longitudinal_disp
  Bus Selector1 : BusSelector  Commented=on  OutputSignals=Longitudinal_vel,Longitudinal_disp,Lateral_vel
  Degrees to Radians : simulink_extras/Transformations/Degrees to Radians
  Demux : Demux  Commented=on  Outputs=3
  From1 : From  Commented=on  GotoTag=Lateral_driver_inputs  TagVisibility=global
  From2 : From  Commented=on  GotoTag=chassisbus  TagVisibility=global
  MATLAB Function : MATLAB Function  Commented=on  TreatAsAtomicUnit=on
  MATLAB Function1 : MATLAB Function  Commented=on  TreatAsAtomicUnit=on
  cmd_str : Outport
  wires:
  From1/1 -> Demux/1
  Demux/1 -> MATLAB Function/1(X)
  Demux/2 -> MATLAB Function/2(Y)
  Demux/3 -> MATLAB Function/3(PSI)
  From2/1 -> Bus Selector1/1
  Bus Selector1/1 -> MATLAB Function/4(vx)  "<Longitudinal_vel>"
  Bus Selector1/2 -> 1-D Lookup Table4/1, 1-D Lookup Table3/1, 1-D Lookup Table2/1  "<Longitudinal_disp>"
  1-D Lookup Table4/1 -> MATLAB Function/8(path_Theta)
  1-D Lookup Table3/1 -> MATLAB Function/7(path_X)
  1-D Lookup Table2/1 -> MATLAB Function/6(path_Y)
  Bus Selector/1 -> 1-D Lookup Table/1  "<Longitudinal_disp>"
  1-D Lookup Table/1 -> Degrees to Radians/1
  [chassisbus] -> Bus Selector/1
  Degrees to Radians/1 -> Add/2
  Bus Selector1/3 -> MATLAB Function/5(vy)  "<Lateral_vel>"
  Add/1 -> cmd_str/1
  MATLAB Function/1(delta) -> Add/1

== system Vehicle_Model_999_Modular_roll_gradient/Inputs/throttle_input_simulink ==
  In1 : Inport
  1-D Lookup Table : Lookup_n-D  Commented=on  NumberOfTableDimensions=1  BreakpointsForDimension1=ctrl_s  Table=ctrl_Throttle  InternalRulePriority=Speed  RndMeth=Simplest
  Bus Selector : BusSelector  Commented=on  OutputSignals=Longitudinal_disp
  Clock : Clock  Commented=on
  Constant : Constant  Commented=on  Value=0.5
  Constant1 : Constant  Commented=on
  From : From  Commented=on  GotoTag=chassisbus  TagVisibility=global
  Switch : Switch  Commented=on  Criteria=u2 > Threshold  Threshold=2  SaturateOnIntegerOverflow=off  InputSameDT=off
  accln_simulink : Outport
  wires:
  From/1 -> Bus Selector/1
  Bus Selector/1 -> 1-D Lookup Table/1  "<Longitudinal_disp>"
  Constant/1 -> Switch/1
  Constant1/1 -> Switch/3
  Clock/1 -> Switch/2
  In1/1 -> accln_simulink/1

== system Vehicle_Model_999_Modular_roll_gradient/Vehicle dynamics/Brakes ==
  Bus Selector : BusSelector  OutputSignals=Brake_input
  Bus Selector1 : BusSelector  OutputSignals=Omega
  Gain : Gain  Commented=on  Gain=100
  MATLAB Function : MATLAB Function  TreatAsAtomicUnit=on
  Terminator : Terminator
  Terminator1 : Terminator
  To Workspace : ToWorkspace  Commented=on  VariableName=Brake_input_percent  SaveFormat=Timeseries  SampleTime=-1
  To Workspace1 : ToWorkspace  Commented=on  VariableName=Front_braking_torque  SaveFormat=Timeseries  SampleTime=-1
  To Workspace2 : ToWorkspace  Commented=on  VariableName=Rear_braking_torque  SaveFormat=Timeseries  SampleTime=-1
  tag scope: Brake_torques=global
  wires:
  MATLAB Function/1(T_brakes) -> [Brake_torques]
  MATLAB Function/2(T_mag_Front) -> Terminator/1, To Workspace1/1  "Front_braking_torque"
  MATLAB Function/3(T_mag_Rear) -> To Workspace2/1, Terminator1/1  "Rear_braking_torque"
  Gain/1 -> To Workspace/1  "brak_pedal_input_percent"
  [Input_bus] -> Bus Selector/1
  Bus Selector/1 -> MATLAB Function/1(brake_pedal), Gain/1  "<Brake_input>"
  [Wheel_bus] -> Bus Selector1/1
  Bus Selector1/1 -> MATLAB Function/2(omega)  "<Omega>"

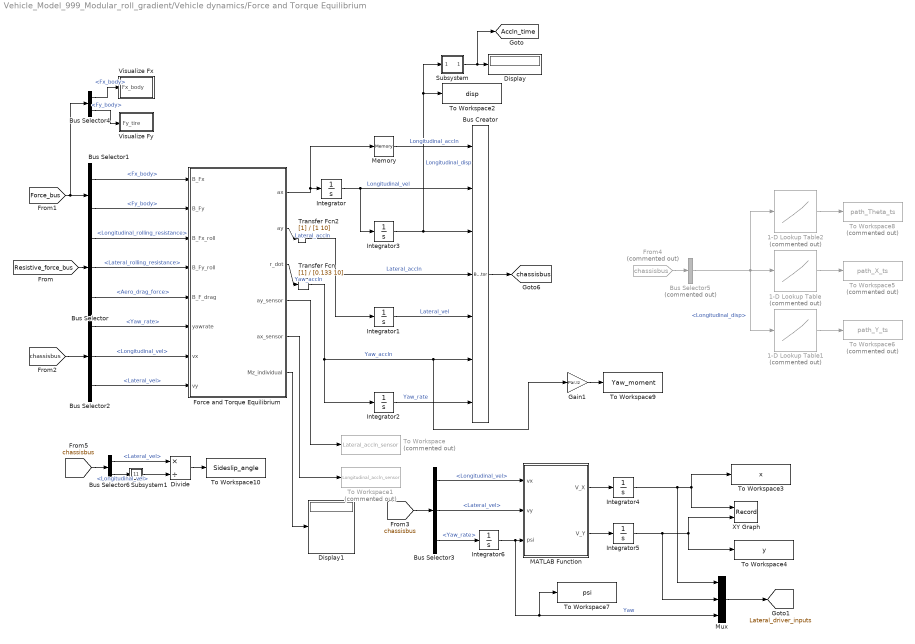
== system Vehicle_Model_999_Modular_roll_gradient/Vehicle dynamics/Force and Torque Equilibrium ==
  1-D Lookup Table : Lookup_n-D  Commented=on  NumberOfTableDimensions=1  BreakpointsForDimension1=ctrl_s  Table=path_X  InternalRulePriority=Speed  RndMeth=Simplest
  1-D Lookup Table1 : Lookup_n-D  Commented=on  NumberOfTableDimensions=1  BreakpointsForDimension1=ctrl_s  Table=path_Y  InternalRulePriority=Speed  RndMeth=Simplest
  1-D Lookup Table2 : Lookup_n-D  Commented=on  NumberOfTableDimensions=1  BreakpointsForDimension1=ctrl_s  Table=path_Theta  InternalRulePriority=Speed  RndMeth=Simplest
  Bus Creator : BusCreator  Inputs=7
  Bus Selector : BusSelector  OutputSignals=Longitudinal_rolling_resistance,Lateral_rolling_resistance,Aero_drag_force
  Bus Selector1 : BusSelector  OutputSignals=Fx_body,Fy_body
  Bus Selector2 : BusSelector  OutputSignals=Yaw_rate,Longitudinal_vel,Lateral_vel
  Bus Selector3 : BusSelector  OutputSignals=Longitudinal_vel,Lateral_vel,Yaw_rate
  Bus Selector4 : BusSelector  OutputSignals=Fx_body,Fy_body
  Bus Selector5 : BusSelector  Commented=on  OutputSignals=Longitudinal_disp
  Bus Selector6 : BusSelector  OutputSignals=Lateral_vel,Longitudinal_vel
  Display : Display
  Display1 : Display
  Divide : Product  Inputs=*/
  Force and Torque Equilibrium : MATLAB Function  TreatAsAtomicUnit=on
  From4 : From  Commented=on  GotoTag=chassisbus  TagVisibility=global
  Gain1 : Gain  Gain=Par.Iz
  Integrator : Integrator  InitialCondition=init_vx  LimitOutput=on  UpperSaturationLimit=1e6  LowerSaturationLimit=0
  Integrator1 : Integrator  InitialCondition=init_vy  LimitOutput=on  UpperSaturationLimit=1e6
  Integrator2 : Integrator  InitialCondition=init_r  LimitOutput=on  UpperSaturationLimit=1e6
  Integrator{3..6} (4 alike) : Integrator
  MATLAB Function : MATLAB Function  TreatAsAtomicUnit=on
  Memory : Memory
  Mux : Mux  Inputs=3
  Subsystem : Subsystem
  Subsystem1 : Subsystem
  To Workspace : ToWorkspace  Commented=on  VariableName=Lateral_accln_sensor  SaveFormat=Timeseries  SampleTime=-1
  To Workspace1 : ToWorkspace  Commented=on  VariableName=Longitudinal_accln_sensor  SaveFormat=Timeseries  SampleTime=-1
  To Workspace10 : ToWorkspace  VariableName=Sideslip_angle  SaveFormat=Timeseries  SampleTime=-1
  To Workspace2 : ToWorkspace  VariableName=disp  SaveFormat=Timeseries  SampleTime=-1
  To Workspace3 : ToWorkspace  VariableName=x  SaveFormat=Timeseries  SampleTime=-1
  To Workspace4 : ToWorkspace  VariableName=y  SaveFormat=Timeseries  SampleTime=-1
  To Workspace5 : ToWorkspace  Commented=on  VariableName=path_X_ts  SaveFormat=Timeseries  SampleTime=-1
  To Workspace6 : ToWorkspace  Commented=on  VariableName=path_Y_ts  SaveFormat=Timeseries  SampleTime=-1
  To Workspace7 : ToWorkspace  VariableName=psi  SaveFormat=Timeseries  SampleTime=-1
  To Workspace8 : ToWorkspace  Commented=on  VariableName=path_Theta_ts  SaveFormat=Timeseries  SampleTime=-1
  To Workspace9 : ToWorkspace  VariableName=Yaw_moment  SaveFormat=Timeseries  SampleTime=-1
  Transfer Fcn : TransferFcn  Denominator=[0.133 10]
  Transfer Fcn2 : TransferFcn  Denominator=[1 10]
  Visualize Fx : Subsystem
      settings: PortSchema="{\"entries\":[{\"content\":{\"sides\":[{\"content\":{},\"type\":\"ConnectorPlacement.EquallySpacedRectSide\",\"uuid\":\"1b308914-9cf8-47f9-8fbc-f2a7158e3eb5\"},{\"content\":{\"side\":\"RIGHT\"},\"type\":\"ConnectorPlacement.EquallySpacedRectSide\",\"uuid\":\"484927c0-b1be-45c4-bf4e-6bbdeba32628\"},{\"content\":{\"side\":\"TOP\"},\"type\":\"ConnectorPlacement.EquallySpacedRectSide\",\"uuid\":\"29e445e7-e31e-448a-ad1b-232db6da9c2a\"},{\"content\":{\"connectorIds\":[\"In1\"],\"side\":\"BOTTOM\"},\"type\":\"ConnectorPlacement.EquallySpacedRectSide\",\"uuid\":\"dd5671a5-30f2-4fe9-831d-0b6bb30f66ee\"}]},\"type\":\"ConnectorPlacement.EquallySpacedConnector\",\"uuid\":\"173edc1f-5f22-4703-a5c3-9a1f8cb52657\"}],\"packageUris\":[\"http://schema.mathworks.com/mf0/Connector/R2020b\"],\"version\":\"1.0\"}"
  Visualize Fy : Subsystem
      settings: PortSchema="{\"entries\":[{\"content\":{\"sides\":[{\"content\":{},\"type\":\"ConnectorPlacement.EquallySpacedRectSide\",\"uuid\":\"1b308914-9cf8-47f9-8fbc-f2a7158e3eb5\"},{\"content\":{\"side\":\"RIGHT\"},\"type\":\"ConnectorPlacement.EquallySpacedRectSide\",\"uuid\":\"484927c0-b1be-45c4-bf4e-6bbdeba32628\"},{\"content\":{\"side\":\"TOP\"},\"type\":\"ConnectorPlacement.EquallySpacedRectSide\",\"uuid\":\"29e445e7-e31e-448a-ad1b-232db6da9c2a\"},{\"content\":{\"connectorIds\":[\"In1\"],\"side\":\"BOTTOM\"},\"type\":\"ConnectorPlacement.EquallySpacedRectSide\",\"uuid\":\"3b440e80-ce08-4e27-92f2-f1f752eee795\"}]},\"type\":\"ConnectorPlacement.EquallySpacedConnector\",\"uuid\":\"173edc1f-5f22-4703-a5c3-9a1f8cb52657\"}],\"packageUris\":[\"http://schema.mathworks.com/mf0/Connector/R2020b\"],\"version\":\"1.0\"}"
  XY Graph : Record  NumPorts=2.0  FileSettingsInternal="{\"entries\":[{\"content\":{\"excelSettings\":{\"content\":{},\"type\":\"Streamout.ExcelSettings\"},\"parquetSettings\":{\"content\":{},\"type\":\"Streamout.ParquetSettings\"}},\"type\":\"Streamout.FileSettingStorage\",\"uuid\":\"\"}],\"packageUris\":[\"http:\\/\\/schema.mathworks.com\\/mf0\\/streamout_blocks\\/R2020a\"],\"version\":\"1.0\"}"  FrameSettings=[0, 0]  Layout=[1 1]  SignalsInternal="{\"entries\":[{\"content\":{\"signals\":[{\"content\":{\"blockPath\":[],\"dimensions\":[1],\"domain\":\"\",\"lineColor\":\"#22b573\",\"lineWidth\":2,\"port\":1,\"sid\":[\"\"],\"signalID\":1,\"signalName\":\"Integrator4\"},\"type\":\"RecordBlkView.Signal\",\"uuid\":\"\"},{\"content\":{\"blockPath\":[],\"dimensions\":[1],\"domain\":\"\",\"lineColor\":\"#0072bd\",\"lineWidth\":2,\"port\":2,\"sid\":[\"\"],\"signalID\":2,\"signalName\":\"Integrator5\"},\"type\":\"RecordBlkView.Signal\",\"uuid\":\"\"}]},\"type\":\"RecordBlkView.InputSignals\",\"uuid\":\"\"}],\"packageUris\":[\"http:\\/\\/schema.mathworks.com\\/mf0\\/streamout_blocks\\/R2020a\"],\"version\":\"1.0\"}"  VisualizationBindings="{\"xyplotplugin\":{\"info\":[{\"series\":[{\"bindingParametersList\":[{\"parameter\":\"X-Axis\",\"signalID\":148193,\"signalName\":\"Integrator4\"},{\"parameter\":\"Y-Axis\",\"signalID\":148197,\"signalName\":\"Integrator5\"}],\"seriesID\":0}],\"subplotID\":1}]}}"  CompatibilityTag=XY
  tag scope: Accln_time=global, Lateral_driver_inputs=global, chassisbus=global
  wires:
  Force and Torque Equilibrium/4(ay_sensor) -> To Workspace/1
  Integrator1/1 -> Bus Creator/5  "Lateral_vel"
  Integrator3/1 -> Subsystem/1(In1), To Workspace2/1, Bus Creator/3  "Longitudinal_disp"
  Bus Creator/1 -> [chassisbus]
  Bus Selector/1 -> Force and Torque Equilibrium/3(B_Fx_roll)  "<Longitudinal_rolling_resistance>"
  Integrator/1 -> Integrator3/1, Bus Creator/2  "Longitudinal_vel"
  Force and Torque Equilibrium/5(ax_sensor) -> To Workspace1/1
  Subsystem/1(Out1) -> [Accln_time], Display/1
  Force and Torque Equilibrium/3(r_dot) -> Transfer Fcn/1  "Yaw_accln"
  [Resistive_force_bus] -> Bus Selector/1
  Bus Selector/2 -> Force and Torque Equilibrium/4(B_Fy_roll)  "<Lateral_rolling_resistance>"
  Bus Selector/3 -> Force and Torque Equilibrium/5(B_F_drag)  "<Aero_drag_force>"
  [Force_bus] -> Bus Selector1/1, Bus Selector4/1
  Bus Selector1/1 -> Force and Torque Equilibrium/1(B_Fx)  "<Fx_body>"
  Bus Selector1/2 -> Force and Torque Equilibrium/2(B_Fy)  "<Fy_body>"
  [chassisbus] -> Bus Selector2/1
  Bus Selector2/1 -> Force and Torque Equilibrium/6(yawrate)  "<Yaw_rate>"
  Bus Selector2/2 -> Force and Torque Equilibrium/7(vx)  "<Longitudinal_vel>"
  Bus Selector2/3 -> Force and Torque Equilibrium/8(vy)  "<Lateral_vel>"
  Integrator2/1 -> Bus Creator/7  "Yaw_rate"
  Force and Torque Equilibrium/1(ax) -> Memory/1, Integrator/1
  Memory/1 -> Bus Creator/1  "Longitudinal_accln"
  Force and Torque Equilibrium/2(ay) -> Transfer Fcn2/1  "Lateral_accln"
  Transfer Fcn/1 -> Gain1/1, Bus Creator/6, Integrator2/1  "Yaw_accln"
  Transfer Fcn2/1 -> Bus Creator/4, Integrator1/1  "Lateral_accln"
  MATLAB Function/1(V_X) -> Integrator4/1
  MATLAB Function/2(V_Y) -> Integrator5/1
  [chassisbus] -> Bus Selector3/1
  Bus Selector3/1 -> MATLAB Function/1(vx)  "<Longitudinal_vel>"
  Bus Selector3/2 -> MATLAB Function/2(vy)  "<Lateral_vel>"
  Bus Selector3/3 -> Integrator6/1  "<Yaw_rate>"
  Integrator6/1 -> Mux/3, To Workspace7/1, MATLAB Function/3(psi)  "Yaw"
  Integrator4/1 -> Mux/1, To Workspace3/1, XY Graph/1
  Integrator5/1 -> Mux/2, To Workspace4/1, XY Graph/2
  Bus Selector4/1 -> Visualize Fx/1(Fx_body)  "<Fx_body>"
  Bus Selector4/2 -> Visualize Fy/1(Fy_tire)  "<Fy_body>"
  Mux/1 -> [Lateral_driver_inputs]
  From4/1 -> Bus Selector5/1
  Bus Selector5/1 -> 1-D Lookup Table1/1, 1-D Lookup Table2/1, 1-D Lookup Table/1  "<Longitudinal_disp>"
  1-D Lookup Table/1 -> To Workspace5/1
  1-D Lookup Table1/1 -> To Workspace6/1
  1-D Lookup Table2/1 -> To Workspace8/1
  Gain1/1 -> To Workspace9/1
  [chassisbus] -> Bus Selector6/1
  Bus Selector6/1 -> Divide/1  "<Lateral_vel>"
  Bus Selector6/2 -> Subsystem1/1(In1)  "<Longitudinal_vel>"
  Subsystem1/1(Out1) -> Divide/2
  Divide/1 -> To Workspace10/1
  Force and Torque Equilibrium/6(Mz_individual) -> Display1/1

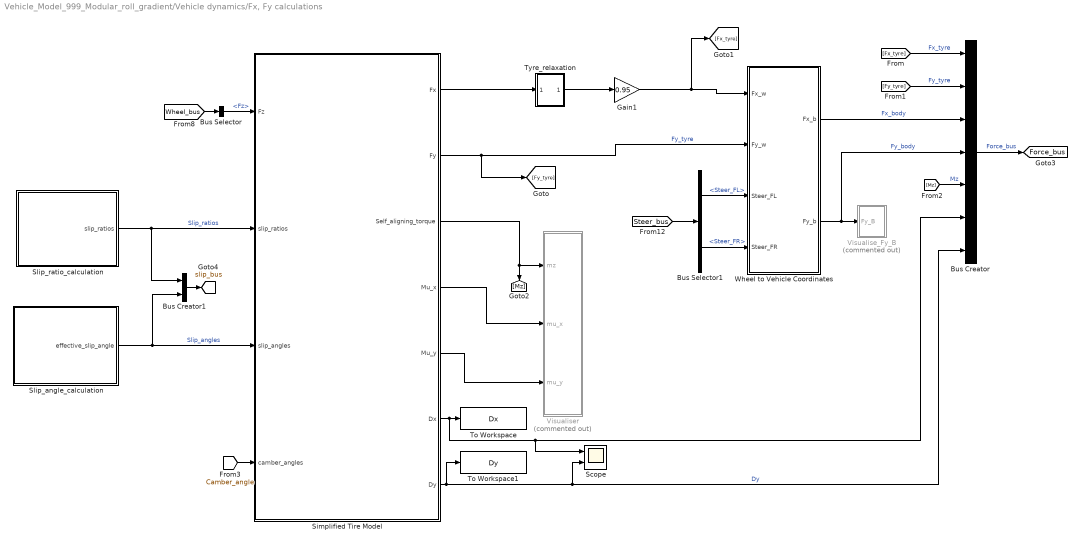
== system Vehicle_Model_999_Modular_roll_gradient/Vehicle dynamics/Fx, Fy calculations ==
  Bus Creator : BusCreator  Inputs=7
  Bus Creator1 : BusCreator  Inputs=2
  Bus Selector : BusSelector  OutputSignals=Fz
  Bus Selector1 : BusSelector  OutputSignals=Steer_FL,Steer_FR
  Gain1 : Gain  Gain=0.95
  Scope : Scope  NumInputPorts=2
      settings: ActiveDisplayYMinimum=-148.8876055299138  ActiveDisplayYMaximum=1339.9884497692244  DataLoggingVariableName=ScopeData3
  Simplified Tire Model : MATLAB Function  TreatAsAtomicUnit=on
  Slip_angle_calculation : Subsystem
  Slip_ratio_calculation : Subsystem
  To Workspace : ToWorkspace  VariableName=Dx  SaveFormat=Timeseries  SampleTime=-1
  To Workspace1 : ToWorkspace  VariableName=Dy  SaveFormat=Timeseries  SampleTime=-1
  Tyre_relaxation : Subsystem
  Visualise_Fy_B : Subsystem  Commented=on
  Visualiser : Subsystem  Commented=on
  Wheel to Vehicle Coordinates : MATLAB Function  TreatAsAtomicUnit=on
  tag scope: Force_bus=global, slip_bus=global
  wires:
  [Camber_angle] -> Simplified Tire Model/4(camber_angles)
  Wheel to Vehicle Coordinates/2(Fy_b) -> Bus Creator/4, Visualise_Fy_B/1(Fy_B)  "Fy_body"
  Simplified Tire Model/3(Self_aligning_torque) -> [Mz], Visualiser/1(mz)
  Tyre_relaxation/1(Fx_w) -> Gain1/1
  Simplified Tire Model/7(Dy) -> To Workspace1/1, Scope/2, Bus Creator/7  "Dy"
  Bus Selector1/1 -> Wheel to Vehicle Coordinates/3(Steer_FL)  "<Steer_FL>"
  Simplified Tire Model/5(Mu_y) -> Visualiser/3(mu_y)
  Simplified Tire Model/2(Fy) -> Wheel to Vehicle Coordinates/2(Fy_w), [Fy_tyre]  "Fy_tyre"
  Wheel to Vehicle Coordinates/1(Fx_b) -> Bus Creator/3  "Fx_body"
  Simplified Tire Model/4(Mu_x) -> Visualiser/2(mu_x)
  [Steer_bus] -> Bus Selector1/1
  Bus Selector1/2 -> Wheel to Vehicle Coordinates/4(Steer_FR)  "<Steer_FR>"
  Gain1/1 -> Wheel to Vehicle Coordinates/1(Fx_w), [Fx_tyre]
  Slip_angle_calculation/1(effective_slip_angle) -> Bus Creator1/2, Simplified Tire Model/3(slip_angles)  "Slip_angles"
  Slip_ratio_calculation/1(slip_ratios) -> Bus Creator1/1, Simplified Tire Model/2(slip_ratios)  "Slip_ratios"
  [Fy_tyre] -> Bus Creator/2  "Fy_tyre"
  [Fx_tyre] -> Bus Creator/1  "Fx_tyre"
  [Mz] -> Bus Creator/5  "Mz"
  Bus Creator/1 -> [Force_bus]  "Force_bus"
  Bus Creator1/1 -> [slip_bus]
  Bus Selector/1 -> Simplified Tire Model/1(Fz)  "<Fz>"
  [Wheel_bus] -> Bus Selector/1
  Simplified Tire Model/6(Dx) -> Scope/1, Bus Creator/6, To Workspace/1
  Simplified Tire Model/1(Fx) -> Tyre_relaxation/1(Fx_ss)

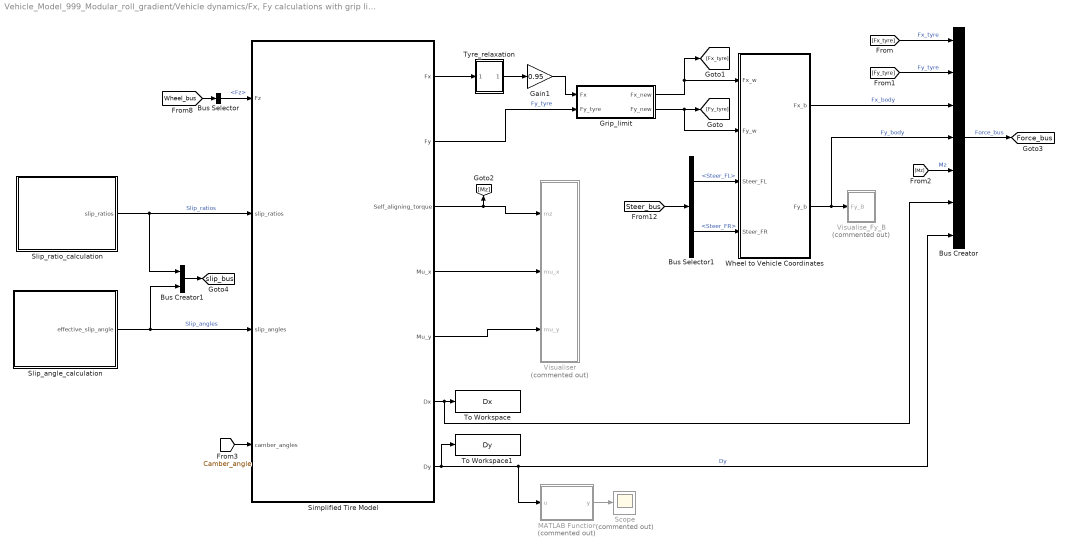
== system Vehicle_Model_999_Modular_roll_gradient/Vehicle dynamics/Fx, Fy calculations with grip limit ==
  Bus Creator : BusCreator  Inputs=7
  Bus Creator1 : BusCreator  Inputs=2
  Bus Selector : BusSelector  OutputSignals=Fz
  Bus Selector1 : BusSelector  OutputSignals=Steer_FL,Steer_FR
  Gain1 : Gain  Gain=0.95
  Grip_limit : Subsystem
  MATLAB Function : MATLAB Function  Commented=on  TreatAsAtomicUnit=on
  Scope : Scope  Commented=on
      settings: ActiveDisplayYMinimum=-1  ActiveDisplayYMaximum=1  DataLoggingVariableName=ScopeData16
  Simplified Tire Model : MATLAB Function  TreatAsAtomicUnit=on
  Slip_angle_calculation : Subsystem
  Slip_ratio_calculation : Subsystem
  To Workspace : ToWorkspace  VariableName=Dx  SaveFormat=Timeseries  SampleTime=-1
  To Workspace1 : ToWorkspace  VariableName=Dy  SaveFormat=Timeseries  SampleTime=-1
  Tyre_relaxation : Subsystem
  Visualise_Fy_B : Subsystem  Commented=on
  Visualiser : Subsystem  Commented=on
  Wheel to Vehicle Coordinates : MATLAB Function  TreatAsAtomicUnit=on
  tag scope: Force_bus=global, slip_bus=global
  wires:
  Simplified Tire Model/1(Fx) -> Tyre_relaxation/1(Fx_ss)
  Simplified Tire Model/6(Dx) -> To Workspace/1, Bus Creator/6
  [Wheel_bus] -> Bus Selector/1
  Bus Selector/1 -> Simplified Tire Model/1(Fz)  "<Fz>"
  Bus Creator1/1 -> [slip_bus]
  Bus Creator/1 -> [Force_bus]  "Force_bus"
  [Mz] -> Bus Creator/5  "Mz"
  [Fx_tyre] -> Bus Creator/1  "Fx_tyre"
  [Fy_tyre] -> Bus Creator/2  "Fy_tyre"
  Slip_ratio_calculation/1(slip_ratios) -> Simplified Tire Model/2(slip_ratios), Bus Creator1/1  "Slip_ratios"
  Slip_angle_calculation/1(effective_slip_angle) -> Simplified Tire Model/3(slip_angles), Bus Creator1/2  "Slip_angles"
  Bus Selector1/2 -> Wheel to Vehicle Coordinates/4(Steer_FR)  "<Steer_FR>"
  [Steer_bus] -> Bus Selector1/1
  Simplified Tire Model/4(Mu_x) -> Visualiser/2(mu_x)
  Wheel to Vehicle Coordinates/1(Fx_b) -> Bus Creator/3  "Fx_body"
  Simplified Tire Model/5(Mu_y) -> Visualiser/3(mu_y)
  Bus Selector1/1 -> Wheel to Vehicle Coordinates/3(Steer_FL)  "<Steer_FL>"
  Simplified Tire Model/7(Dy) -> MATLAB Function/1(u), Bus Creator/7, To Workspace1/1  "Dy"
  Tyre_relaxation/1(Fx_w) -> Gain1/1
  Simplified Tire Model/3(Self_aligning_torque) -> Visualiser/1(mz), [Mz]
  Wheel to Vehicle Coordinates/2(Fy_b) -> Visualise_Fy_B/1(Fy_B), Bus Creator/4  "Fy_body"
  [Camber_angle] -> Simplified Tire Model/4(camber_angles)
  MATLAB Function/1(y) -> Scope/1
  Grip_limit/2(Fy_new) -> Wheel to Vehicle Coordinates/2(Fy_w), [Fy_tyre]
  Grip_limit/1(Fx_new) -> [Fx_tyre], Wheel to Vehicle Coordinates/1(Fx_w)
  Gain1/1 -> Grip_limit/1(Fx)
  Simplified Tire Model/2(Fy) -> Grip_limit/2(Fy_tyre)  "Fy_tyre"
